simulink model "ServoModel_v0"  (R2021b)
settings: Solver=FixedStepAuto  StartTime=0.0  StopTime=100  RelTol=1e-3  EnableMultiTasking=on
libraries: simulink x1, arduinolib x1
settings Model: ExtModeTrigDuration=2  Creator=diego  LastModifiedBy=diego
settings OptimizationCC: EnhancedBackFolding=on  PassReuseOutputArgsAs=Individual arguments  ZeroExternalMemoryAtStartup=off  ZeroInternalMemoryAtStartup=off  MaxStackSize=64  OptimizeBlockOrder=speed  DifferentSizesBufferReuse=on  EfficientTunableParamExpr=on
settings DebuggingCC: ParameterTunabilityLossMsg=error
settings HardwareCC: ProdBitPerInt=16  ProdBitPerPointer=16  ProdBitPerSizeT=16  ProdBitPerPtrDiffT=16  ProdLargestAtomicFloat=None  ProdWordSize=8  ProdHWDeviceType=Atmel->AVR
settings SFSimCC: MATLABDynamicMemAlloc=off
settings RTWCC: Description=Embedded Coder  SystemTargetFile=ert.tlc  HardwareBoard=Arduino Uno  TemplateMakefile=ert_default_tmf  Toolchain=Arduino AVR  BuildConfiguration=Faster Runs
settings CodeAppCC: ForceParamTrailComments=on  IgnoreCustomStorageClasses=off  OperatorAnnotations=on  SimulinkDataObjDesc=on  SFDataObjDesc=on  InsertBlockDesc=on
settings ERTTargetCC: SupportContinuousTime=on  SupportVariableSizeSignals=on  ExtModeTransport=3  ExtModeStaticAlloc=on  ExtModeStaticAllocSize=250  ExtModeMexFile=ext_xcp  ExtModeIntrfLevel=Level2 - Open

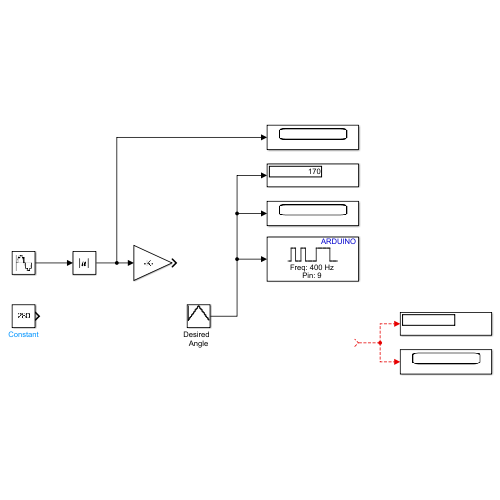
[thumbnail: Simulink's stored preview of the top-level diagram]
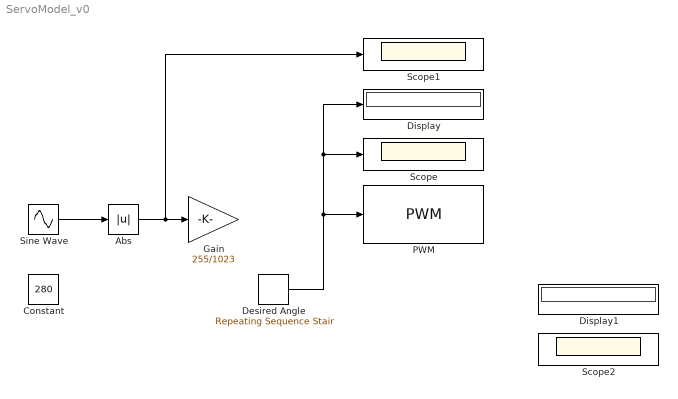
== system ServoModel_v0 ==
  Abs : Abs
  Constant : Constant  Value=280
  Desired Angle : simulink/Sources/Repeating Sequence Stair  OutValues=[60:255 254:-1:61]  tsamp=0.005  OutMin=[0]  OutMax=[255]  OutDataTypeStr=uint8  OutputDataTypeScalingMode=uint8  OutDataType=fixdt(0,8)  ConRadixGroup=Best Precision: Vector-wise  OutScaling=2^-12
  Display : Display
  Display1 : Display
  Gain : Gain  Gain=255/1023
  PWM : arduinolib/PWM  pinNumber=9  frequencyType=Specify  desiredFrequency=400  achievableFrequency=400
  Scope : Scope
  Scope1 : Scope
  Scope2 : Scope
  Sine Wave : Sin  Amplitude=1023  SampleTime=0.01
  wires:
  Abs/1 -> Scope1/1, Gain/1
  Sine Wave/1 -> Abs/1
  ? -> Scope2/1, Display1/1
  Desired Angle/1 -> Display/1, Scope/1, PWM/1
